simulink model "AveragePerEpoch"  (R2016b)
settings: Solver=FixedStepAuto  StartTime=0.0  StopTime=inf  FixedStep=sCoreParams.core.stepPeriod*50  RelTol=1e-3  SampleTimeConstraint=STIndependent  EnableMultiTasking=on
undefined symbols (not defined in the file): neuralModelParams, sCoreParams
libraries: dspstat3 x1
settings Model: Creator=anish  LastModifiedBy=rzelmann
settings SolverCC: EnableConcurrentExecution=on  AutoInsertRateTranBlk=on
settings DataIOCC: SaveFormat=StructureWithTime  SignalLoggingSaveFormat=ModelDataLogs  SaveOutput=off  SignalLogging=off  DSMLogging=off  SaveTime=off
settings OptimizationCC: BlockReduction=off  ConditionallyExecuteInputs=off  DefaultParameterBehavior=Inlined  OptimizeBlockIOStorage=off  BufferReuse=off  GlobalBufferReuse=off  ExpressionFolding=off  LocalBlockOutputs=off  LifeSpan=inf
settings DebuggingCC: SignalRangeChecking=error  SaveWithParameterizedLinksMsg=none  AllowSymbolicDim=off  ModelReferenceSymbolNameMessage=none  StateNameClashWarn=warning  SFUnexpectedBacktrackingDiag=warning  SFNoUnconditionalDefaultTransitionDiag=warning  SFExecutionAtInitializationDiag=none
settings HardwareCC: ProdBitPerPointer=32  ProdBitPerSizeT=32  ProdBitPerPtrDiffT=32  ProdLargestAtomicFloat=None  ProdWordSize=32  ProdLongLongMode=on  ProdHWDeviceType=Generic->32-bit x86 compatible  TargetBitPerPointer=64  TargetLargestAtomicFloat=Float  TargetLongLongMode=on  TargetIntDivRoundTo=Zero  TargetEndianess=LittleEndian  TargetWordSize=64  TargetHWDeviceType=Intel->x86-64 (Windows64)
settings ModelReferenceCC: UpdateModelReferenceTargets=Force  ModelReferenceNumInstancesAllowed=Single  ModelReferencePassRootInputsByReference=off
settings RTWCC: SystemTargetFile=slrt.tlc  TemplateMakefile=slrt_default_tmf  Description=Simulink Real-Time  BuildConfiguration=Faster Runs  RTWCompilerOptimization=on
settings ConfigComp: CovMetricSettings=dw  CovHtmlReporting=on  CovSaveCumulativeToWorkspaceVar=on  CovSaveSingleToWorkspaceVar=on  CovExternalEMLEnable=off  CovSFcnEnable=off

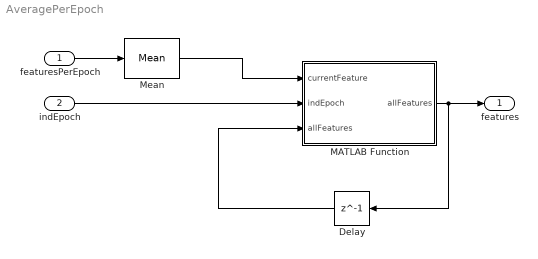
== system AveragePerEpoch ==
  featuresPerEpoch : Inport  PortDimensions=[floor(sCoreParams.decoders.txDetector.detectionDurationSteps / neuralModelParams.nEpochs) neuralModelParams.nFeaturesPerEpoch]
  indEpoch : Inport  Port=2
  Delay : Delay  DelayLength=1  InitialCondition=zeros(1, neuralModelParams.nFeatures)
  MATLAB Function : MATLAB Function  TreatAsAtomicUnit=on
  Mean : dspstat3/Mean  run=off  reset_popup=None  InputProcessing=Columns as channels (frame based)  directionMode=Each column  dimension=1  roiEnable=off  roiType=Rectangles  roiPortion=Entire ROI  roiOutput=Individual statistics for each ROI  roiFlag=off  outputDataTypeStr=Inherit: Same as accumulator  outputLastDataTypeStr=Inherit: Same as accumulator  outputMin=[]  outputMax=[]  roundingMode=Floor  overflowMode=off
  features : Outport
  wires:
  MATLAB Function/1(allFeatures) -> features/1, Delay/1
  featuresPerEpoch/1 -> Mean/1
  indEpoch/1 -> MATLAB Function/2(indEpoch)
  Delay/1 -> MATLAB Function/3("allFeatures ")
  Mean/1 -> MATLAB Function/1(currentFeature)

== matlab function AveragePerEpoch/MATLAB Function ==
  data: currentFeature input; indEpoch input; allFeatures input; allFeatures output
function allFeatures = organizeFeaturesPerEpoch(currentFeature, indEpoch, allFeatures)

lFeat = length(currentFeature);
%if (indEpoch*lFeat<=size(allFeatures,1) % changed to not sending the trigger signal to start with
allFeatures((indEpoch-1)*lFeat+1:indEpoch*lFeat, 1) = currentFeature;
%end
